simulink model "CLSfixedExample2"  (R2025b)
settings: Solver=FixedStepAuto  StartTime=0.0  StopTime=4  FixedStep=0.0005  RelTol=1e-3
undefined symbols (not defined in the file): AVI, cfg_length, LRI, pNode_length, pPath_length, PulsePeriod, PVARP, stepsize, URI, VRP
libraries: Libs x7, Libs_unified x6
settings Model: SimulationMode=accelerator  Creator=ball907  LastModifiedBy=rfen801
settings SolverCC: EnableFixedStepZeroCrossing=on

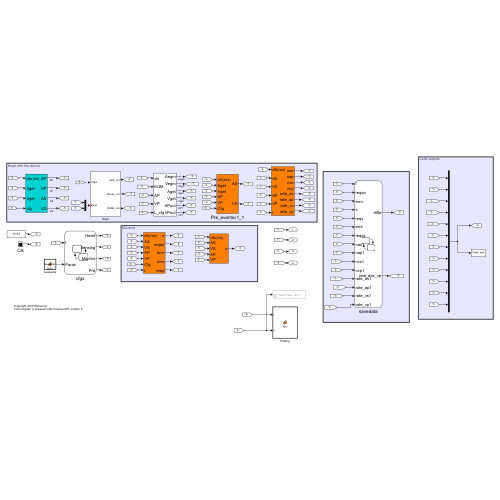
[thumbnail: Simulink's stored preview of the top-level diagram]
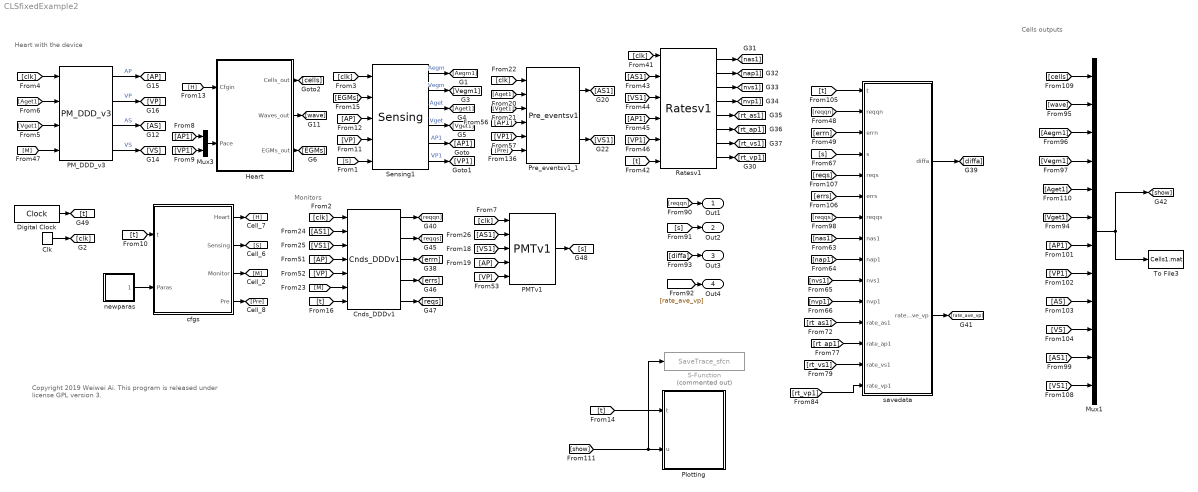
== system CLSfixedExample2 ==
  note: Cells outputs
  note: Copyright 2019 Weiwei Ai.
      | This program is released under license GPL version 3.
  note: Heart with the device
  note: Monitors
  Clk : DiscretePulseGenerator  PulseType=Time based  Period=1  PulseWidth=50
  Cnds_DDDv1 : Libs_unified/Cnds_DDDv1  SystemSampleTime=-1  VariantActivationTime=update diagram  EmptyChoice=off  PassThrough=off  PassThroughVariantControl=(default)  EmptyChoiceVariantControl=(default)  AllowFlexibleInterface=on  Latency=0  AutoFrameSizeCalculation=off
  Digital Clock : DigitalClock  SampleTime=stepsize
  Heart : Subsystem
  Mux1 : Mux  Inputs=12
  Mux3 : Mux  Inputs=2
  PMTv1 : Libs_unified/PMTv1  SystemSampleTime=-1  VariantActivationTime=update diagram  EmptyChoice=off  PassThrough=off  PassThroughVariantControl=(default)  EmptyChoiceVariantControl=(default)  AllowFlexibleInterface=on  Latency=0  AutoFrameSizeCalculation=off
  PM_DDD_v3 : Libs_unified/PM_DDD_v3  SystemSampleTime=-1  VariantActivationTime=update diagram  EmptyChoice=off  PassThrough=off  PassThroughVariantControl=(default)  EmptyChoiceVariantControl=(default)  AllowFlexibleInterface=on  Latency=0  AutoFrameSizeCalculation=off
  Plotting : MATLAB Function  TreatAsAtomicUnit=on  SystemSampleTime=stepsize*5
  Pre_eventsv1_1 : Libs_unified/Pre_eventsv1  SystemSampleTime=-1  VariantActivationTime=update diagram  EmptyChoice=off  PassThrough=off  PassThroughVariantControl=(default)  EmptyChoiceVariantControl=(default)  AllowFlexibleInterface=on  Latency=0  AutoFrameSizeCalculation=off
  Ratesv1 : Libs_unified/Ratesv1  SystemSampleTime=-1  VariantActivationTime=update diagram  EmptyChoice=off  PassThrough=off  PassThroughVariantControl=(default)  EmptyChoiceVariantControl=(default)  AllowFlexibleInterface=on  Latency=0  AutoFrameSizeCalculation=off
  S-Function : S-Function  Commented=on  FunctionName=SaveTrace_sfcn  Parameters=1  SFunctionDeploymentMode=off  EnableBusSupport=off
  Sensing1 : Libs_unified/Sensing  SystemSampleTime=-1  VariantActivationTime=update diagram  EmptyChoice=off  PassThrough=off  PassThroughVariantControl=(default)  EmptyChoiceVariantControl=(default)  AllowFlexibleInterface=on  Latency=0  AutoFrameSizeCalculation=off
  To File3 : ToFile  Filename=Cells1.mat  MatrixName=cells
      settings: Decimation=2
  cfgs : Stateflow chart  TreatAsAtomicUnit=on
  newparas : MATLAB Function  TreatAsAtomicUnit=on
  savedata : Stateflow chart  TreatAsAtomicUnit=on
  Out1 : Outport
  Out2 : Outport  Port=2
  Out3 : Outport  Port=3
  Out4 : Outport  Port=4
  wires:
  Ratesv1/4 -> [nvp1]
  [reqqn] -> Out1/1
  [Vget1] -> PM_DDD_v3/3
  [VP] -> Sensing1/4
  [AS1] -> Ratesv1/2
  Sensing1/1 -> [Aegm1]  "Aegm"
  [AP1] -> Mux1/7
  PM_DDD_v3/2 -> [VP]  "VP"
  [rt_as1] -> savedata/12(rate_as1)
  Ratesv1/3 -> [nvs1]
  [reqs] -> savedata/5(reqs)
  [t] -> Ratesv1/6
  Ratesv1/2 -> [nap1]
  [AS1] -> Cnds_DDDv1/2
  [AS] -> Mux1/9
  Sensing1/3 -> [Aget1]  "Aget"
  [AS1] -> PMTv1/2
  [M] -> PM_DDD_v3/4
  [s] -> Out2/1
  [VP1] -> Ratesv1/5
  [AP1] -> Mux3/1
  [VP1] -> Pre_eventsv1_1/5
  [t] -> savedata/1(t)
  savedata/1(diffa) -> [diffa]
  Cnds_DDDv1/1 -> [reqqn]
  [AP1] -> Ratesv1/4
  [AP] -> Sensing1/3
  [nap1] -> savedata/9(nap1)
  Sensing1/6 -> [VP1]  "VP1"
  Sensing1/5 -> [AP1]  "AP1"
  PMTv1/1 -> [s]
  [M] -> Cnds_DDDv1/6
  [AP1] -> Pre_eventsv1_1/4
  [s] -> savedata/4(s)
  Heart/3(EGMs_out) -> [EGMs]
  [diffa] -> Out3/1
  [cells] -> Mux1/1
  Cnds_DDDv1/4 -> [errs]
  Ratesv1/7 -> [rt_vs1]
  [clk] -> PM_DDD_v3/1
  Sensing1/4 -> [Vget1]  "Vget"
  Pre_eventsv1_1/1 -> [AS1]
  [EGMs] -> Sensing1/2
  [Vget1] -> Mux1/6
  [VP1] -> Mux1/8
  [VS1] -> Cnds_DDDv1/3
  [clk] -> Sensing1/1
  Ratesv1/6 -> [rt_ap1]
  [S] -> Sensing1/5
  Digital Clock/1 -> [t]
  [AP] -> PMTv1/4
  [nas1] -> savedata/8(nas1)
  [reqqn] -> savedata/2(reqqn)
  Clk/1 -> [clk]
  [VS] -> Mux1/10
  [nvp1] -> savedata/11(nvp1)
  Cnds_DDDv1/3 -> [errn]
  Ratesv1/5 -> [rt_as1]
  Sensing1/2 -> [Vegm1]  "Vegm"
  [H] -> Heart/1(Cfgin)
  Cnds_DDDv1/2 -> [reqqs]
  [VS1] -> PMTv1/3
  [AS1] -> Mux1/11
  [Aget1] -> Pre_eventsv1_1/2
  [errs] -> savedata/6(errs)
  PM_DDD_v3/3 -> [AS]  "AS"
  [clk] -> PMTv1/1
  Pre_eventsv1_1/2 -> [VS1]
  [rt_vp1] -> savedata/15(rate_vp1)
  [VS1] -> Mux1/12
  Ratesv1/1 -> [nas1]
  [VP] -> PMTv1/5
  [clk] -> Ratesv1/1
  PM_DDD_v3/4 -> [VS]  "VS"
  savedata/2(rate_ave_vp) -> [rate_ave_vp]
  [rt_ap1] -> savedata/13(rate_ap1)
  [Aegm1] -> Mux1/3
  [t] -> Cnds_DDDv1/7
  [reqqs] -> savedata/7(reqqs)
  [rate_ave_vp] -> Out4/1
  Cnds_DDDv1/5 -> [reqs]
  [VP] -> Cnds_DDDv1/5
  [VP1] -> Mux3/2
  ? -> ?
  [clk] -> Pre_eventsv1_1/1
  Heart/1(Cells_out) -> [cells]
  [errn] -> savedata/3(errn)
  [rt_vs1] -> savedata/14(rate_vs1)
  [Aget1] -> Mux1/5
  [Pre] -> Pre_eventsv1_1/6
  [VS1] -> Ratesv1/3
  PM_DDD_v3/1 -> [AP]  "AP"
  Mux1/1 -> [show], To File3/1
  [nvs1] -> savedata/10(nvs1)
  [Vget1] -> Pre_eventsv1_1/3
  [Vegm1] -> Mux1/4
  [AP] -> Cnds_DDDv1/4
  Heart/2(Waves_out) -> [wave]
  [wave] -> Mux1/2
  Ratesv1/8 -> [rt_vp1]
  [Aget1] -> PM_DDD_v3/2
  [clk] -> Cnds_DDDv1/1
  cfgs/2(Sensing) -> [S]
  cfgs/4(Pre) -> [Pre]
  newparas/1(newparas) -> cfgs/2(Paras)
  cfgs/3(Monitor) -> [M]
  cfgs/1(Heart) -> [H]
  [t] -> cfgs/1(t)
  [show] -> S-Function/1, Plotting/2(u)
  [t] -> Plotting/1(t)
  Mux3/1 -> Heart/2(Pace)

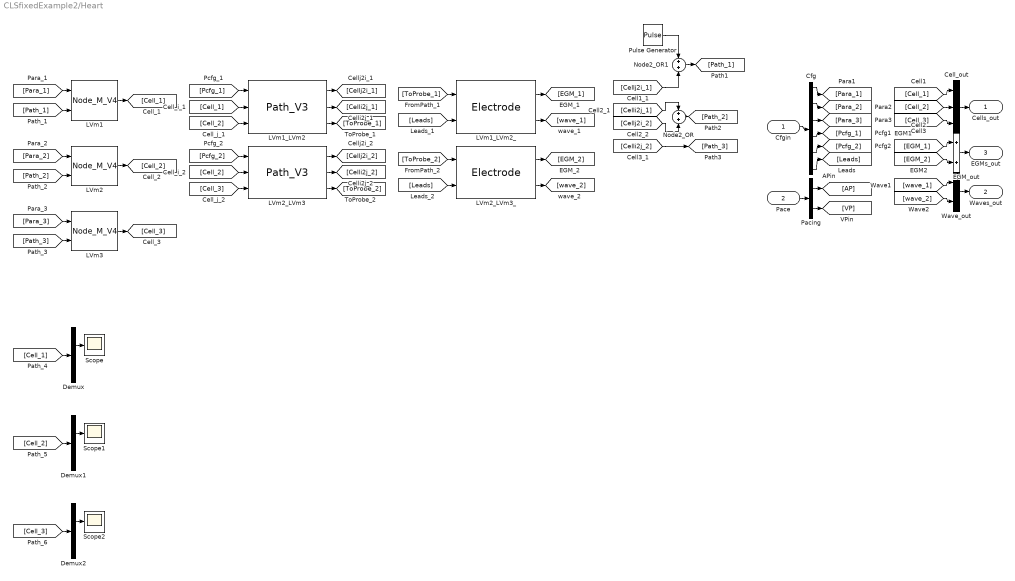
== system CLSfixedExample2/Heart ==
  Cfgin : Inport
  Pace : Inport  Port=2
  Cell_out : Mux  Inputs=3
  Cfg : Demux  Outputs=[25,25,25,11,11,28]
  Demux : Demux  Outputs=5
  Demux1 : Demux  Outputs=5
  Demux2 : Demux  Outputs=5
  EGM_out : Sum  Inputs=2
  LVm1 : Libs/Node_M_V4  SystemSampleTime=-1  VariantActivationTime=update diagram  EmptyChoice=off  PassThrough=off  PassThroughVariantControl=(default)  EmptyChoiceVariantControl=(default)  AllowFlexibleInterface=on  Latency=0  AutoFrameSizeCalculation=off
  LVm1_LVm2 : Libs/Path_V3  SystemSampleTime=-1  VariantActivationTime=update diagram  EmptyChoice=off  PassThrough=off  PassThroughVariantControl=(default)  EmptyChoiceVariantControl=(default)  AllowFlexibleInterface=on  Latency=0  AutoFrameSizeCalculation=off
  LVm1_LVm2_ : Libs/Electrode  SystemSampleTime=-1  VariantActivationTime=update diagram  EmptyChoice=off  PassThrough=off  PassThroughVariantControl=(default)  EmptyChoiceVariantControl=(default)  AllowFlexibleInterface=on  Latency=0  AutoFrameSizeCalculation=off
  LVm2 : Libs/Node_M_V4  SystemSampleTime=-1  VariantActivationTime=update diagram  EmptyChoice=off  PassThrough=off  PassThroughVariantControl=(default)  EmptyChoiceVariantControl=(default)  AllowFlexibleInterface=on  Latency=0  AutoFrameSizeCalculation=off
  LVm2_LVm3 : Libs/Path_V3  SystemSampleTime=-1  VariantActivationTime=update diagram  EmptyChoice=off  PassThrough=off  PassThroughVariantControl=(default)  EmptyChoiceVariantControl=(default)  AllowFlexibleInterface=on  Latency=0  AutoFrameSizeCalculation=off
  LVm2_LVm3_ : Libs/Electrode  SystemSampleTime=-1  VariantActivationTime=update diagram  EmptyChoice=off  PassThrough=off  PassThroughVariantControl=(default)  EmptyChoiceVariantControl=(default)  AllowFlexibleInterface=on  Latency=0  AutoFrameSizeCalculation=off
  LVm3 : Libs/Node_M_V4  SystemSampleTime=-1  VariantActivationTime=update diagram  EmptyChoice=off  PassThrough=off  PassThroughVariantControl=(default)  EmptyChoiceVariantControl=(default)  AllowFlexibleInterface=on  Latency=0  AutoFrameSizeCalculation=off
  Node2_OR : Sum  Inputs=2
  Node2_OR1 : Sum  Inputs=2
  Pacing : Demux  Outputs=2
  Pulse Generator : DiscretePulseGenerator  PulseType=Time based  Amplitude=120  Period=PulsePeriod  PulseWidth=20
  Scope : Scope
  Scope1 : Scope
  Scope2 : Scope
      settings: DataLoggingVariableName=ScopeData2
  Wave_out : Mux  Inputs=2
  Cells_out : Outport
  Waves_out : Outport  Port=2
  EGMs_out : Outport  Port=3
  wires:
  [wave_2] -> Wave_out/2
  [wave_1] -> Wave_out/1
  [EGM_2] -> EGM_out/2
  [EGM_1] -> EGM_out/1
  [Cell_3] -> Cell_out/3
  [Cell_2] -> Cell_out/2
  [Cell_1] -> Cell_out/1
  Wave_out/1 -> Waves_out/1
  EGM_out/1 -> EGMs_out/1
  Cell_out/1 -> Cells_out/1
  Pacing/2 -> [VP]
  Pacing/1 -> [AP]
  Cfg/6 -> [Leads]
  Cfg/5 -> [Pcfg_2]
  Cfg/4 -> [Pcfg_1]
  Cfg/3 -> [Para_3]
  Cfg/2 -> [Para_2]
  Cfg/1 -> [Para_1]
  Pace/1 -> Pacing/1
  Cfgin/1 -> Cfg/1
  [Celli2j_2] -> [Path_3]
  Node2_OR/1 -> [Path_2]
  [Cellj2i_2] -> Node2_OR/2
  [Celli2j_1] -> Node2_OR/1
  [Leads] -> LVm2_LVm3_/2
  [ToProbe_2] -> LVm2_LVm3_/1
  LVm2_LVm3_/2 -> [wave_2]
  LVm2_LVm3_/1 -> [EGM_2]
  [Leads] -> LVm1_LVm2_/2
  [ToProbe_1] -> LVm1_LVm2_/1
  LVm1_LVm2_/2 -> [wave_1]
  LVm1_LVm2_/1 -> [EGM_1]
  [Cell_3] -> LVm2_LVm3/3
  [Cell_2] -> LVm2_LVm3/2
  [Pcfg_2] -> LVm2_LVm3/1
  LVm2_LVm3/3 -> [ToProbe_2]
  LVm2_LVm3/2 -> [Celli2j_2]
  LVm2_LVm3/1 -> [Cellj2i_2]
  [Cell_2] -> LVm1_LVm2/3
  [Cell_1] -> LVm1_LVm2/2
  [Pcfg_1] -> LVm1_LVm2/1
  LVm1_LVm2/3 -> [ToProbe_1]
  LVm1_LVm2/2 -> [Celli2j_1]
  LVm1_LVm2/1 -> [Cellj2i_1]
  [Path_3] -> LVm3/2
  [Para_3] -> LVm3/1
  LVm3/1 -> [Cell_3]
  [Path_2] -> LVm2/2
  [Para_2] -> LVm2/1
  LVm2/1 -> [Cell_2]
  [Path_1] -> LVm1/2
  [Para_1] -> LVm1/1
  LVm1/1 -> [Cell_1]
  [Cell_1] -> Demux/1
  Demux/2 -> Scope/1
  Demux1/2 -> Scope1/1
  [Cell_2] -> Demux1/1
  Demux2/2 -> Scope2/1
  [Cell_3] -> Demux2/1
  Node2_OR1/1 -> [Path_1]
  [Cellj2i_1] -> Node2_OR1/2
  Pulse Generator/1 -> Node2_OR1/1

== stateflow chart CLSfixedExample2/cfgs ==
  settings: executeAtInitialization=1
  state Ini
  state wait
  Ini -> wait : [t>800]{pUpdate(Paras);}
  (default) -> Ini : {Sensing=Scfgf;[Monitor, Pre]=Precfg;...
      |  [Heart] =LoadInit;}
  data: Scfg function_output; Mcfg function_output; Preout function_output; LRI parameter; AVI parameter; VRP parameter; URI parameter; PVARP parameter; Parasin function_input; pNode_length parameter; pPath_length parameter; Hcfg function_output; cfg_length parameter; Heart output; Sensing output; Monitor output; t input; Paras input; Pre output
  function Scfg= Scfgf:
    | function Scfg= Scfgf
    | 
    | %% desired
    | xa=1;
    | xc=0.05;
    | xc1=0.1;
    | xd=1;
    | xe=0.1;
    | avd=100;
    | vad=100;
    | uni_a=1;
    | Sens_a=0.6;
    | Amp_ap=500;
    | uni_v=1;
    | Sens_v=2.8;
    | Amp_vp=500;
    | 
    | Scfg=[xa xc xc1 xd xe avd vad uni_a Sens_a Amp_ap uni_v Sens_v Amp_vp]';
    | 
    | end
  function [Mcfg,Preout]= Precfg:
    | function [Mcfg,Preout]= Precfg
    | % 
    | % LRI=1000;
    | % AVI=170;
    | % URI=500;
    | % VRP=230;
    | % PVARP=250;
    | Mcfg=[LRI AVI URI VRP PVARP];
    | Preout=[VRP PVARP];
    | 
    | end
  function pUpdate(Parasin):
    | %% Get the index of the parameter
    | function pUpdate(Parasin)
    | %#codegen
    | coder.extrinsic('evalin');
    | coder.extrinsic('assignin');
    | Nodein=zeros(1,pNode_length); % The total number of cell cfg ports
    | Nodein=evalin('base', 'pNode');
    | Pathin=zeros(1,pPath_length); % The total number of path cfg ports
    | Pathin=evalin('base', 'pPath');
    | for n=1:pNode_length
    |     m=Nodein(n);
    |     Heart(m)=Parasin(n);
    | end
    | 
    | for n=1:pPath_length
    |     m=Pathin(n);
    |     nn=n+length(Nodein);
    |     Heart(m)=Parasin(nn);
    | end
    | 
    | assignin('base', 'Params', Parasin);
    | 
    | end
  function Hcfg   = LoadInit:
    | function Hcfg   = LoadInit
    | %#codegen
    | coder.extrinsic('evalin');
    | Hcfg1=zeros(1,cfg_length); % The total number of cfg ports
    | Hcfg1=evalin('base', 'cfgdata');
    | Hcfg=Hcfg1';
    | end

== matlab function CLSfixedExample2/Plotting ==
  data: t input; u input
function fcn(t,u)
%coder.extrinsic('evalin')
coder.extrinsic('updateGUIplots')
fun = 'updateGUIplots';
updateGUIplots(t,u)
%feval(fun,t,u)
end

== matlab function CLSfixedExample2/newparas ==
  data: newparas output; paras_length parameter

function newparas= auto(paras_length)

coder.extrinsic('evalin');
%par_length = evalin('base','paras_length')
newparas=zeros(1,paras_length); % The total number of cell cfg ports
newparas=evalin('base', 'pp');

end

== stateflow chart CLSfixedExample2/savedata ==
  settings: executeAtInitialization=1
  state termi
  state difa
  state Ini
  difa -> termi [order 1] : [rate_ave_a0>=60]/{coder.extrinsic('assignin');diffa=rate_ave_a1-rate_ave_a0;assignin('base', 'diffa', diffa);}
  (default) -> Ini : {rate_ave_vp=0; diffa=0;smax=0;}
  Ini -> difa [order 1] : [t>=29998]{coder.extrinsic('assignin','mean');assignin('base', 'reqqn', reqqn);assignin('base', 'errn', errn);assignin('base', 'smax', smax);...
      | assignin('base', 'errs', errs);assignin('base', 'reqs', reqs);assignin('base', 'reqqs', reqqs);...
      | assignin('base', 'nas1', nas1);assignin('base', 'nap1', nap1);assignin('base', 'nvs1', nvs1);assignin('base', 'nvp1', nvp1);...
      | assignin('base', 'rate_as1', rate_as1);assignin('base', 'rate_ap1', rate_ap1);assignin('base', 'rate_vs1', rate_vs1);assignin('base', 'rate_vp1', rate_vp1);...
      | rate_ave_vp=mean(rate_vp1(2,1:nvp1));assignin('base', 'rate_ave_vp', rate_ave_vp);...
      | rate_ave_a1=0;rate_ave_a1=mean([rate_as1(2,1:nas1) ]);rate_ave_a0=0;rate_ave_a0=zeros(size(rate_ave_a1),like=rate_ave_a1);}
  difa -> termi [order 2] : [rate_ave_a0<60]/{coder.extrinsic('assignin');diffa=rate_ave_a1-60;assignin('base', 'diffa', diffa);}
  Ini -> Ini [order 2] : [s>smax]/{smax=s;}
  data: t input; reqqn input; errn input; s input; reqs input; errs input; reqqs input; nas1 input; nap1 input; nvs1 input; nvp1 input; rate_as1 input; rate_ap1 input; rate_vs1 input; rate_vp1 input; diffa output double; rate_ave_a1 local double; rate_ave_vp output double; rate_ave_a0 local double; smax local
